simulink model "untitled"  (R2014a)
settings: Solver=ode45  StartTime=0.0  StopTime=10.0  RelTol=1e-3
libraries: powerlib_meascontrol x1
settings Model: Creator=ztg  LastModifiedBy=ztg

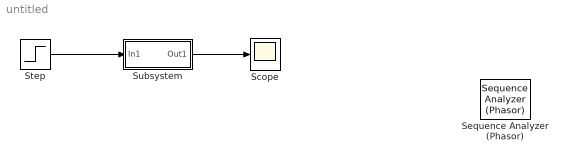
== system untitled ==
  Scope : Scope
  Sequence Analyzer (Phasor) : powerlib_meascontrol/Measurements/Sequence Analyzer (Phasor)  seq=Positive
  Step : Step  SampleTime=0
  Subsystem : Subsystem
  wires:
  Step/1 -> Subsystem/1(In1)
  Subsystem/1(Out1) -> Scope/1

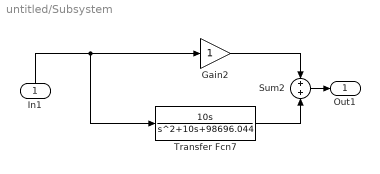
== system untitled/Subsystem ==
  In1 : Inport
  Gain2 : Gain
  Sum2 : Sum
  Transfer Fcn7 : TransferFcn  Numerator=[10 0]  Denominator=[1 10 98696.044]
  Out1 : Outport
  wires:
  Gain2/1 -> Sum2/1
  Transfer Fcn7/1 -> Sum2/2
  In1/1 -> Transfer Fcn7/1, Gain2/1
  Sum2/1 -> Out1/1
